simulink model "mavsim_chap13_gimbal"  (Simulink 8.8)
settings: Solver=ode45  StartTime=0.0  StopTime=400  RelTol=1e-3  EnableMultiTasking=on
undefined symbols (not defined in the file or in its folder): autopilot, camera, drawEnvironmentCamera, estimate_states, forces_moments, gps, map, P, path_follow, path_manager, path_planner, point_gimbal, sensors, true_states
libraries: simulink x4
settings Model: SuppressorTable=22 serialization::archive 11 0 3 0 0 0 11 0  Creator=beard  LastModifiedBy=nathan
settings OptimizationCC: ExpressionDepthLimit=2147483647  InitFltsAndDblsToZero=on
settings DebuggingCC: SolverPrmCheckMsg=warning  StrictBusMsg=Warning
settings SFSimCC: SimParseCustomCode=off

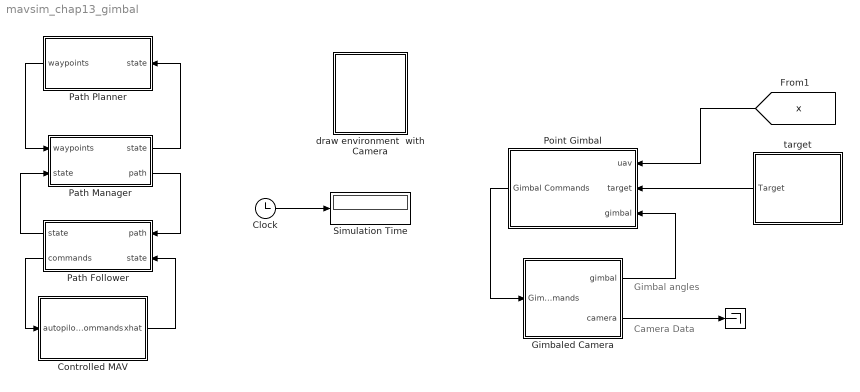
== system mavsim_chap13_gimbal ==
  note: Gimbal angles
  note: Camera Data
  " " : Terminator
  Clock : Clock
  Controlled MAV : Subsystem
      mask Display: image(imread('batcam.png'))
  Gimbaled Camera : Subsystem
      mask Display: image(imread('gimbal.jpg'))
  Path Follower : Subsystem
  Path Manager : Subsystem
  Path Planner : Subsystem
  Point Gimbal : Subsystem
  Simulation Time : Display
  draw environment  with Camera : Subsystem  mask{map=map, R_min=P.R_min, cam_fov=P.cam_fov}
      mask prompts: cam_fov "FOV of Camera"
      mask init:
      | % parameters for drawing aircraft
      |   % scale size
      |   size = 1;
      |   fuse_l1    = 7;
      |   fuse_l2    = 4;
      |   fuse_l3    = 15;
      |   fuse_w     = 2;
      |   wing_l     = 6;
      |   wing_w     = 20;
      |   tail_l     = 3;
      |   tail_h     = 3;
      |   tailwing_w = 10;
      |   tailwing_l = 3;
      |   % colors
      |   red     = [1, 0, 0];
      |   green   = [0, 1, 0];
      |   blue    = [0, 0, 1];
      |   yellow  = [1,1,0];
      |   magenta = [0, 1, 1];
      |   
      | 
      | % define vertices and faces for aircraft
      |   V = [...
      |     fuse_l1,             0,             0;...        % point 1
      |     fuse_l2,            -fuse_w/2,     -fuse_w/2;... % point 2     
      |     fuse_l2,             fuse_w/2,     -fuse_w/2;... % point 3     
      |     fuse_l2,             fuse_w/2,      fuse_w/2;... % point 4
      |     fuse_l2,            -fuse_w/2,      fuse_w/2;... % point 5
      |    -fuse_l3,             0,             0;...        % point 6
      |     0,                   wing_w/2,      0;...        % point 7
      |    -wing_l,              wing_w/2,      0;...        % point 8
      |    -wing_l,             -wing_w/2,      0;...        % point 9
      |     0,                  -wing_w/2,      0;...        % point 10
      |    -fuse_l3+tailwing_l,  tailwing_w/2,  0;...        % point 11
      |    -fuse_l3,             tailwing_w/2,  0;...        % point 12
      |    -fuse_l3,            -tailwing_w/2,  0;...        % point 13
      |    -fuse_l3+tailwing_l, -tailwing_w/2,  0;...        % point 14
      |    -fuse_l3+tailwing_l,  0,             0;...        % point 15
      |    -fuse_l3+tailwing_l,  0,             -tail_h;...  % point 16
      |    -fuse_l3,             0,             -tail_h;...  % point 17
      |   ];
      |   
      |   F = [...
      |         1,  2,  3,  1;... % nose-top
      |         1,  3,  4,  1;... % nose-left
      |         1,  4,  5,  1;... % nose-bottom
      |         1,  5,  2,  1;... % nose-right
      |         2,  3,  6,  2;... % fuselage-top
      |         3,  6,  4,  3;... % fuselage-left
      |         4,  6,  5,  4;... % fuselage-bottom
      |         2,  5,  6,  2;... % fuselage-right
      |         7,  8,  9, 10;... % wing
      |        11, 12, 13, 14;... % tailwing
      |         6, 15, 17, 17;... % tail
      |         
      |   ];  
      |   
      |   colors = [...
      |         yellow;... % nose-top
      |         yellow;... % nose-left
      |         yellow;... % nose-bottom
      |         yellow;... % nose-right
      |         blue;... % fuselage-top
      |         blue;... % fuselage-left
      |         red;... % fuselage-bottom
      |         blue;... % fuselage-right
      |         green;... % wing
      |         green;... % tailwing
      |         blue;... % tail
      |     ];
      | 
      |   V = size*V;   % rescale vertices
      mask Display: image(imread('tv.jpg'))
  target : Subsystem
      mask Display: image(imread('monstertruck.jpg'))
  wires:
  Clock/1 -> Simulation Time/1
  Path Manager/2(path) -> Path Follower/1(path)
  Path Follower/2(commands) -> Controlled MAV/1(autopilot commands)
  Controlled MAV/1(xhat) -> Path Follower/2(state)
  Path Follower/1("state ") -> Path Manager/2(state)
  Path Manager/1("state ") -> Path Planner/1(state)
  Path Planner/1(waypoints) -> Path Manager/1(waypoints)
  Point Gimbal/1(Gimbal Commands) -> Gimbaled Camera/1(Gimbal Commands)
  Gimbaled Camera/1(gimbal) -> Point Gimbal/3(gimbal)
  target/1(Target) -> Point Gimbal/2(target)
  Gimbaled Camera/2(camera) -> " "/1
  [x] -> Point Gimbal/1(uav)

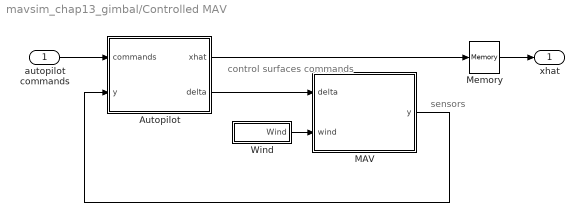
== system mavsim_chap13_gimbal/Controlled MAV ==
  note: sensors
  note: control surfaces
      | commands
  autopilot commands : Inport
  Autopilot : Subsystem
      mask Display: image(imread('kestrel.jpg'))
  MAV : Subsystem
      mask Display: image(imread('batcam.png'))
  Memory : Memory
  Wind : Subsystem
  xhat : Outport
  wires:
  Wind/1(Wind) -> MAV/2(wind)
  Autopilot/2(delta) -> MAV/1(delta)
  MAV/1(y) -> Autopilot/2(y)
  autopilot commands/1 -> Autopilot/1(commands)
  Autopilot/1(xhat) -> Memory/1
  Memory/1 -> xhat/1

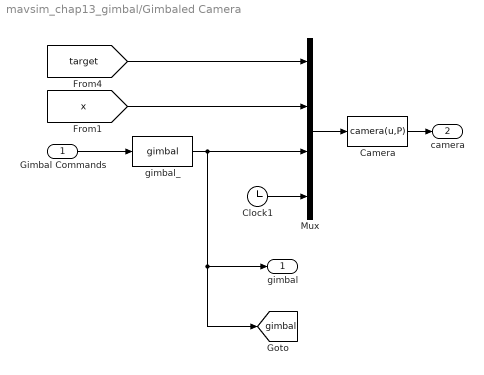
== system mavsim_chap13_gimbal/Gimbaled Camera ==
  Gimbal Commands : Inport
  Camera : MATLABFcn  MATLABFcn=camera(u,P)  OutputDimensions=3  SampleTime=1/P.cam_fps
  Clock1 : Clock
  Mux : Mux
  gimbal_ : S-Function  FunctionName=gimbal  Parameters=P  SFunctionDeploymentMode=off  EnableBusSupport=off
  gimbal : Outport
  camera : Outport  Port=2
  tag scope: gimbal=global
  wires:
  Mux/1 -> Camera/1
  [x] -> Mux/2
  Camera/1 -> camera/1
  [target] -> Mux/1
  Clock1/1 -> Mux/4
  Gimbal Commands/1 -> gimbal_/1
  gimbal_/1 -> Mux/3, gimbal/1, [gimbal]

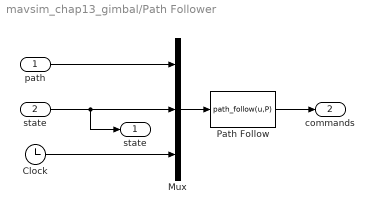
== system mavsim_chap13_gimbal/Path Follower ==
  path : Inport
  state : Inport  Port=2
  Clock : Clock
  Mux : Mux  Inputs=3
  Path Follow : MATLABFcn  MATLABFcn=path_follow(u,P)  OutputDimensions=3  SampleTime=P.Ts
  "state " : Outport
  commands : Outport  Port=2
  wires:
  Path Follow/1 -> commands/1
  Mux/1 -> Path Follow/1
  path/1 -> Mux/1
  Clock/1 -> Mux/3
  state/1 -> Mux/2, "state "/1

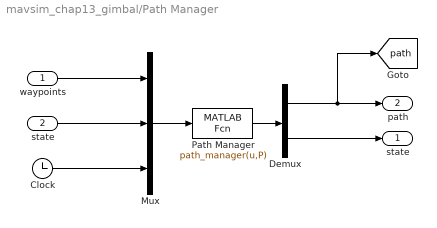
== system mavsim_chap13_gimbal/Path Manager ==
  waypoints : Inport
  state : Inport  Port=2
  Clock : Clock
  Demux : Demux  Outputs=[13;17]
  Mux : Mux  Inputs=3
  Path Manager : MATLABFcn  MATLABFcn=path_manager(u,P)  OutputDimensions=30  SampleTime=P.Ts
  "state " : Outport
  path : Outport  Port=2
  tag scope: path=global
  wires:
  Demux/2 -> "state "/1
  Demux/1 -> [path], path/1
  Path Manager/1 -> Demux/1
  waypoints/1 -> Mux/1
  state/1 -> Mux/2
  Clock/1 -> Mux/3
  Mux/1 -> Path Manager/1

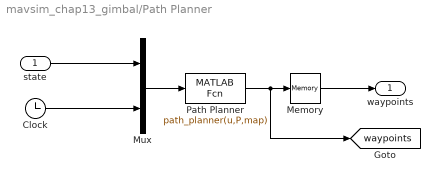
== system mavsim_chap13_gimbal/Path Planner ==
  state : Inport
  Clock : Clock
  Memory : Memory
  Mux : Mux  Inputs=2
  Path Planner : MATLABFcn  MATLABFcn=path_planner(u,P,map)  OutputDimensions=1+5*P.size_waypoint_array  SampleTime=100*P.Ts
  waypoints : Outport
  tag scope: waypoints=global
  wires:
  Mux/1 -> Path Planner/1
  Clock/1 -> Mux/2
  state/1 -> Mux/1
  Path Planner/1 -> Memory/1, [waypoints]
  Memory/1 -> waypoints/1

== system mavsim_chap13_gimbal/Point Gimbal ==
  uav : Inport
  target : Inport  Port=2
  gimbal : Inport  Port=3
  Mux : Mux  Inputs=3
  Point Gimbal : MATLABFcn  MATLABFcn=point_gimbal(u,P)  OutputDimensions=2  SampleTime=P.Ts
  Gimbal Commands : Outport
  wires:
  Mux/1 -> Point Gimbal/1
  uav/1 -> Mux/2
  Point Gimbal/1 -> Gimbal Commands/1
  target/1 -> Mux/1
  gimbal/1 -> Mux/3

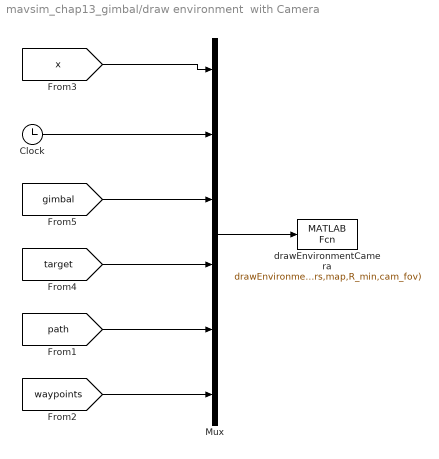
== system mavsim_chap13_gimbal/draw environment  with Camera ==
  Clock : Clock
  Mux : Mux  Inputs=6
  drawEnvironmentCamera : MATLABFcn  MATLABFcn=drawEnvironmentCamera(u,V,F,colors,map,R_min,cam_fov)  OutputDimensions=0  SampleTime=0.1
  wires:
  Clock/1 -> Mux/2
  [x] -> Mux/1
  Mux/1 -> drawEnvironmentCamera/1
  [path] -> Mux/5
  [waypoints] -> Mux/6
  [gimbal] -> Mux/3
  [target] -> Mux/4

== system mavsim_chap13_gimbal/target ==
  S-Function : S-Function  FunctionName=target_motion  Parameters=P,map  SFunctionDeploymentMode=off  EnableBusSupport=off
  Target : Outport
  tag scope: target=global
  wires:
  S-Function/1 -> [target], Target/1

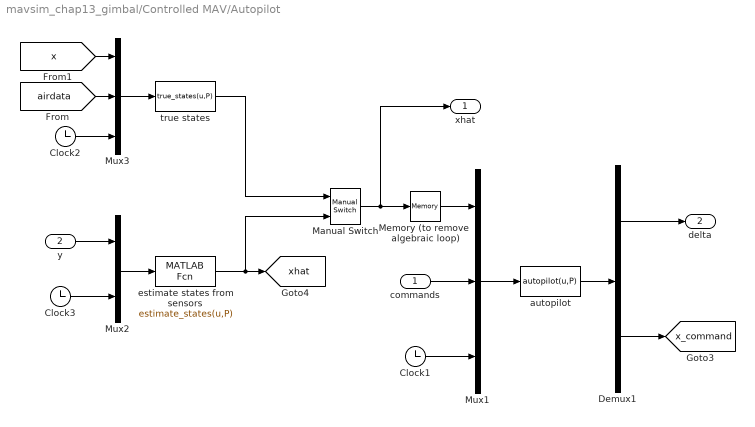
== system mavsim_chap13_gimbal/Controlled MAV/Autopilot ==
  commands : Inport
  y : Inport  Port=2
  Clock1 : Clock
  Clock2 : Clock
  Clock3 : Clock
  Demux1 : Demux  Outputs=[4;12]
  Manual Switch : simulink/Signal Routing/Manual Switch  SystemSampleTime=-1  sw=0  action=0  varsize=off
  Memory (to remove  algebraic loop) : Memory
  Mux1 : Mux  Inputs=3
  Mux2 : Mux  Inputs=2
  Mux3 : Mux  Inputs=3
  autopilot : MATLABFcn  MATLABFcn=autopilot(u,P)  OutputDimensions=4+12  SampleTime=P.Ts
  estimate states from sensors : MATLABFcn  MATLABFcn=estimate_states(u,P)  OutputDimensions=16  SampleTime=P.Ts
  true states : MATLABFcn  MATLABFcn=true_states(u,P)  OutputDimensions=16  SampleTime=P.Ts
  xhat : Outport
  delta : Outport  Port=2
  tag scope: x_command=global, xhat=global
  wires:
  Mux1/1 -> autopilot/1
  autopilot/1 -> Demux1/1
  Demux1/1 -> delta/1
  Demux1/2 -> [x_command]
  commands/1 -> Mux1/2
  Mux2/1 -> estimate states from sensors/1
  y/1 -> Mux2/1
  Memory (to remove  algebraic loop)/1 -> Mux1/1
  Manual Switch/1 -> Memory (to remove  algebraic loop)/1, xhat/1
  true states/1 -> Manual Switch/1
  Mux3/1 -> true states/1
  [airdata] -> Mux3/2
  [x] -> Mux3/1
  Clock1/1 -> Mux1/3
  Clock2/1 -> Mux3/3
  Clock3/1 -> Mux2/2
  estimate states from sensors/1 -> Manual Switch/2, [xhat]

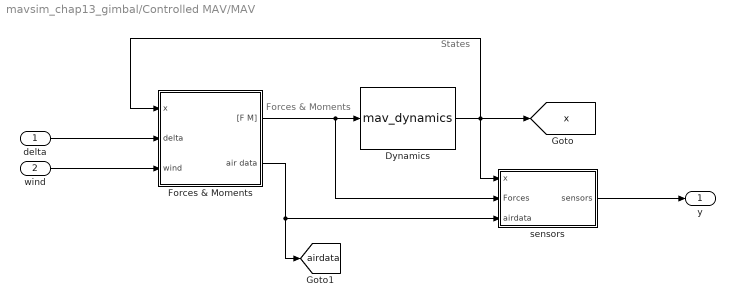
== system mavsim_chap13_gimbal/Controlled MAV/MAV ==
  note: Forces & Moments
  note: States
  delta : Inport
  wind : Inport  Port=2
  Dynamics : S-Function  FunctionName=mav_dynamics  Parameters=mass,Jx,Jy,Jz,Jxz,pn0,pe0,pd0,u0,v0,w0,phi0,theta0,psi0,p0,q0,r0  SFunctionDeploymentMode=off  EnableBusSupport=off  mask{mass=P.mass, Jx=P.Jx, Jy=P.Jy, Jz=P.Jz, Jxz=P.Jxz, pn0=P.pn0, pe0=P.pe0, pd0=P.pd0, u0=P.u0, v0=P.v0, w0=P.w0, phi0=P.phi0, theta0=P.theta0, psi0=P.psi0, p0=P.p0, q0=P.q0, r0=P.r0}
      mask prompts: pn0 "Initial North position"; pe0 "Initial East position"; pd0 "Initial Down position"; u0 "Initial velocy u0"; v0 "Initial velocity v0"; w0 "Initial velocity w0"; phi0 "Initial roll angle"; theta0 "Initial pitch angle"; psi0 "Initial yaw angle"; p0 "Initial roll rate"; q0 "Initial pitch rate"; r0 "Initial yaw rate"
  Forces & Moments : Subsystem
  sensors : Subsystem
  y : Outport
  tag scope: airdata=global, x=global
  wires:
  Dynamics/1 -> sensors/1(x), Forces & Moments/1(x), [x]
  Forces & Moments/1("[F M]") -> sensors/2(Forces), Dynamics/1
  Forces & Moments/2(air data) -> sensors/3(airdata), [airdata]
  delta/1 -> Forces & Moments/2(delta)
  wind/1 -> Forces & Moments/3(wind)
  sensors/1(sensors) -> y/1

== system mavsim_chap13_gimbal/Controlled MAV/Wind ==
  Constant1 : Constant  Value=[0; 0; 0]
  Constant2 : Constant  Value=[P.wind_n; P.wind_e; P.wind_d]
  Mux1 : Mux  Inputs=2
  Wind Gusts : Subsystem
  Wind : Outport
  wires:
  Constant2/1 -> Mux1/1
  Mux1/1 -> Wind/1
  Constant1/1 -> Mux1/2

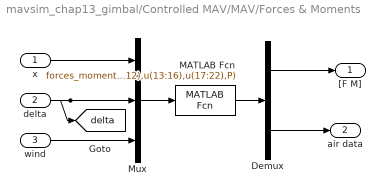
== system mavsim_chap13_gimbal/Controlled MAV/MAV/Forces & Moments ==
  x : Inport
  delta : Inport  Port=2
  wind : Inport  Port=3
  Demux : Demux  Outputs=[6;6]
  MATLAB Fcn : MATLABFcn  MATLABFcn=forces_moments(u(1:12),u(13:16),u(17:22),P)  OutputDimensions=12
  Mux : Mux  Inputs=3
  "[F M]" : Outport
  air data : Outport  Port=2
  tag scope: delta=global
  wires:
  Demux/2 -> air data/1
  Mux/1 -> MATLAB Fcn/1
  Demux/1 -> "[F M]"/1
  MATLAB Fcn/1 -> Demux/1
  wind/1 -> Mux/3
  delta/1 -> [delta], Mux/2
  x/1 -> Mux/1

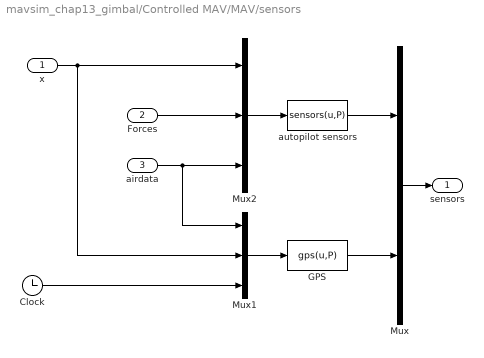
== system mavsim_chap13_gimbal/Controlled MAV/MAV/sensors ==
  x : Inport
  Forces : Inport  Port=2
  airdata : Inport  Port=3
  Clock : Clock
  GPS : MATLABFcn  MATLABFcn=gps(u,P)  OutputDimensions=5  SampleTime=P.Ts_gps
  Mux : Mux  Inputs=2
  Mux1 : Mux  Inputs=3
  Mux2 : Mux  Inputs=3
  autopilot sensors : MATLABFcn  MATLABFcn=sensors(u,P)  OutputDimensions=8  SampleTime=P.Ts
  sensors : Outport
  wires:
  x/1 -> Mux1/2, Mux2/1
  Mux/1 -> sensors/1
  airdata/1 -> Mux1/1, Mux2/3
  Forces/1 -> Mux2/2
  Mux2/1 -> autopilot sensors/1
  Clock/1 -> Mux1/3
  Mux1/1 -> GPS/1
  GPS/1 -> Mux/2
  autopilot sensors/1 -> Mux/1

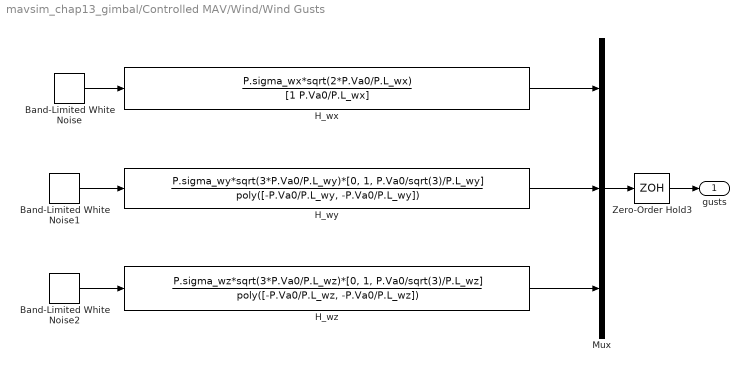
== system mavsim_chap13_gimbal/Controlled MAV/Wind/Wind Gusts ==
  Band-Limited White Noise : simulink/Sources/Band-Limited White Noise  SystemSampleTime=-1  Cov=[1]  Ts=P.Ts  seed=[23341]
  Band-Limited White Noise1 : simulink/Sources/Band-Limited White Noise  SystemSampleTime=-1  Cov=[1]  Ts=P.Ts  seed=[23341]
  Band-Limited White Noise2 : simulink/Sources/Band-Limited White Noise  SystemSampleTime=-1  Cov=[1]  Ts=P.Ts  seed=[23341]
  H_wx : TransferFcn  Numerator=P.sigma_wx*sqrt(2*P.Va0/P.L_wx)  Denominator=[1 P.Va0/P.L_wx]
  H_wy : TransferFcn  Numerator=P.sigma_wy*sqrt(3*P.Va0/P.L_wy)*[0, 1, P.Va0/sqrt(3)/P.L_wy]  Denominator=poly([-P.Va0/P.L_wy, -P.Va0/P.L_wy])
  H_wz : TransferFcn  Numerator=P.sigma_wz*sqrt(3*P.Va0/P.L_wz)*[0, 1, P.Va0/sqrt(3)/P.L_wz]  Denominator=poly([-P.Va0/P.L_wz, -P.Va0/P.L_wz])
  Mux : Mux  Inputs=3
  Zero-Order Hold3 : ZeroOrderHold  SampleTime=P.Ts
  gusts : Outport
  wires:
  H_wx/1 -> Mux/1
  Band-Limited White Noise/1 -> H_wx/1
  H_wy/1 -> Mux/2
  Band-Limited White Noise1/1 -> H_wy/1
  H_wz/1 -> Mux/3
  Band-Limited White Noise2/1 -> H_wz/1
  Mux/1 -> Zero-Order Hold3/1
  Zero-Order Hold3/1 -> gusts/1
